simulink library "MedusaPremix"  (R2022b)
settings: Solver=VariableStepAuto  StartTime=0.0  StopTime=10.0  RelTol=1e-3
values from neighbouring files (symbols this model uses):
  PremixConfig = struct('sample_rate_in_hertz', sample_rate_in_hertz,                            'frame_size', frame_size,                            'rgain_SILENT_GAIN', rgain_SILENT_GAIN,                            'granularity', internal_granularity,                            'LR_in', LR_in, 'LR_out', LR_out,                            'CS_in', CS_in, 'CS_out', CS_out,                            'NumCenterOut' ...(+550 chars)    [MedusaPremixInit.m]
  PremixTune = MedusaPremixTuneInit(tuneFileName, headrestTuneFileName, overheadTuneFileName, MedusaParams)    [MedusaPremixInit.m]    (also in MedusaPremixTuneInit.m = load(tuneFileName))
undefined symbols (not defined in the file or in its folder): carModel, mode, MSConfig, Row
libraries: TuneVar x286, TOP x202, dspmtrx3 x146, FeaturePath x86, matrix_library x20, PooliirLib x8, Pooliir x4
(part 8 of 22)

== system MedusaPremix/Premix51WithMonoSurroundAndCae/Full Mixing Matrix_Center Surround/Fader Downmix ==
  note: downmix
  Front Fade Gain : Inport
  Back Fade Gain : Inport  Port=2
  In Bus Element : Inport  Port=3  PortName=Tuned Inputs  Element=Forward Downmix Threshold
  In Bus Element1 : Inport  Port=3  PortName=Tuned Inputs  Element=Forward Downmix Max
  In Bus Element2 : Inport  Port=3  PortName=Tuned Inputs  Element=Backward Downmix Threshold
  In Bus Element3 : Inport  Port=3  PortName=Tuned Inputs  Element=Backward Downmix Max
  In Bus Element4 : Inport  Port=3  PortName=Tuned Inputs  Element=Downmix Weights CS
  In Bus Element5 : Inport  Port=3  PortName=Tuned Inputs  Element=Downmix Weights CS CAE
  CAE_Enable : Inport  Port=4
  Trigger : TriggerPort  TriggerType=function-call  VariantControl=Variant  PortDimensions=1
  Fading Backward : Subsystem  TreatAsAtomicUnit=on
  Fading Forward : Subsystem  TreatAsAtomicUnit=on
  FeaturePath : FeaturePath/FeaturePath  FeatureName=Fade  IsGroup=off  GroupNumber=-1  DeclarePackages=off  PackageNames=mode,carModel  IsToolGroup=off  TriggerInit=[920 94 1035 201]
      settings: SourceProductName=Bose Talaria
  If : If  NumInputs=2  IfExpression=u1 >= u2
  MATLAB Function : MATLAB Function  TreatAsAtomicUnit=on
  Matrix Multiply : Product
  Merge : Merge
  Downmix : Outport  VectorParamsAs1DForOutWhenUnconnected=off
  DownmixingMatrix : Outport  Port=2  VectorParamsAs1DForOutWhenUnconnected=off
  wires:
  In Bus Element4/1 -> MATLAB Function/1(weights)
  In Bus Element5/1 -> MATLAB Function/2(weights_CAE)
  MATLAB Function/1(downmixWeights) -> Matrix Multiply/2
  In Bus Element3/1 -> Fading Backward/3(backwardDownmixMax)
  In Bus Element2/1 -> Fading Backward/2(backwardDownmixThreshold)
  In Bus Element1/1 -> Fading Forward/3(forwardDownmixMax)
  In Bus Element/1 -> Fading Forward/2(forwardDownmixThreshold)
  If/2 -> Fading Backward/Action
  Fading Forward/1(downmix) -> Merge/1
  Matrix Multiply/1 -> DownmixingMatrix/1
  Back Fade Gain/1 -> If/2, Fading Forward/1(backFadeGain)
  Merge/1 -> Downmix/1, Matrix Multiply/1
  Front Fade Gain/1 -> Fading Backward/1(frontFadeGain), If/1
  Fading Backward/1(downmix) -> Merge/2
  If/1 -> Fading Forward/Action
  CAE_Enable/1 -> MATLAB Function/3(CAE_Enable)

== system MedusaPremix/Premix51WithMonoSurroundAndCae/Full Mixing Matrix_Center Surround/Premixing ==
  Audio Channel Inputs : Inport
  Target Gain : Inport  Port=2
  Matrix Multiply1 : Product  Multiplication=Matrix(*)
  Transpose1 : Math  Operator=transpose  SignedPower=on
  Output : Outport  VectorParamsAs1DForOutWhenUnconnected=off
  wires:
  Matrix Multiply1/1 -> Output/1
  Audio Channel Inputs/1 -> Matrix Multiply1/1
  Target Gain/1 -> Transpose1/1
  Transpose1/1 -> Matrix Multiply1/2

== system MedusaPremix/Premix51WithMonoSurroundAndCae/Full Mixing Matrix_Center Surround/Surround Level Control ==
  RST Trigger : Inport
  SLC Request Trigger : Inport  Port=2
  In Bus Element : Inport  Port=3  PortName=Control Inputs  Element=surround_index
  In Bus Element1 : Inport  Port=3  PortName=Control Inputs  Element=ramp_db_per_second
  In Bus Element2 : Inport  Port=3  PortName=Control Inputs  Element=ramp_milliseconds
  Check Done : Inport  Port=4
  In Bus Element3 : Inport  Port=5  PortName=Tuned Inputs  Element=Min Level CS
  In Bus Element4 : Inport  Port=5  PortName=Tuned Inputs  Element=Detent Level CS
  In Bus Element5 : Inport  Port=5  PortName=Tuned Inputs  Element=Max Level CS
  In Bus Element6 : Inport  Port=5  PortName=Tuned Inputs  Element=Interpolation Method
  In Bus Element7 : Inport  Port=5  PortName=Tuned Inputs  Element=Min Level CS CAE
  In Bus Element8 : Inport  Port=5  PortName=Tuned Inputs  Element=Detent Level CS CAE
  In Bus Element9 : Inport  Port=5  PortName=Tuned Inputs  Element=Max Level CS CAE
  Data Store Memory3 : DataStoreMemory  DataStoreName=Premix_targetGain_CS  ReadBeforeWriteMsg=warning  WriteAfterWriteMsg=warning  WriteAfterReadMsg=warning  InitialValue=1e-5*ones(MedusaPremixConfig.CS_out,MedusaPremixConfig.CS_in)  ShowAdditionalParam=off  OutDataTypeStr=single
  Data Store Memory4 : DataStoreMemory  DataStoreName=Premix_currentGain_CS  ReadBeforeWriteMsg=warning  WriteAfterWriteMsg=warning  WriteAfterReadMsg=warning  InitialValue=1e-5*ones(MedusaPremixConfig.CS_out,MedusaPremixConfig.CS_in)  ShowAdditionalParam=off  OutDataTypeStr=single
  Data Store Read1 : DataStoreRead  DataStoreName=Premix_currentGain_CS  IndexOptions=Index vector (dialog)  Indices=1  OutputSizes=1
  FeaturePath : FeaturePath/FeaturePath  FeatureName=SLC  IsGroup=off  GroupNumber=-1  DeclarePackages=off  PackageNames=mode,carModel  IsToolGroup=off  TriggerInit=[955 319 1070 426]
      settings: SourceProductName=Bose Talaria
  Function-Call Split : FunctionCallSplit  IconShape=distinctive  NumOutputPorts=2
  Initialization and RMDL : MATLAB Function  TreatAsAtomicUnit=on
  Ramper : Subsystem
  Target Gain Computation : MATLAB Function  TreatAsAtomicUnit=on
  Gain Out : Outport  VectorParamsAs1DForOutWhenUnconnected=off
  Ramping Done : Outport  Port=2  VectorParamsAs1DForOutWhenUnconnected=off
  wires:
  In Bus Element9/1 -> Target Gain Computation/6(maxGain_CS_CAE), Initialization and RMDL/6(maxGain_CS_CAE)
  In Bus Element8/1 -> Target Gain Computation/4(detentGain_CS_CAE), Initialization and RMDL/4(detentGain_CS_CAE)
  In Bus Element7/1 -> Target Gain Computation/2(minGain_CS_CAE), Initialization and RMDL/2(minGain_CS_CAE)
  In Bus Element/1 -> Target Gain Computation/9(surr_level), Initialization and RMDL/9(surr_level)
  In Bus Element1/1 -> Ramper/3(ramp rate)
  In Bus Element2/1 -> Ramper/4(ramp time)
  In Bus Element4/1 -> Target Gain Computation/3(detentGain_CS), Initialization and RMDL/3(detentGain_CS)
  In Bus Element3/1 -> Target Gain Computation/1(minGain_CS), Initialization and RMDL/1(minGain_CS)
  In Bus Element6/1 -> Target Gain Computation/7(interpolation_method), Initialization and RMDL/7(interpolation_method)
  In Bus Element5/1 -> Target Gain Computation/5(maxGain_CS), Initialization and RMDL/5(maxGain_CS)
  Ramper/1(ramping done) -> Ramping Done/1
  SLC Request Trigger/1 -> Function-Call Split/1
  Function-Call Split/2 -> Ramper/1(RTC Recv Trigger)
  Function-Call Split/1 -> Target Gain Computation/Trigger
  Target Gain Computation/1(gain_out) -> Ramper/2(target gains (linear))
  Check Done/1 -> Ramper/5(check sequence trigger)
  RST Trigger/1 -> Initialization and RMDL/Trigger
  Data Store Read1/1 -> Gain Out/1
  [CAE_Enable] -> Initialization and RMDL/8(CAE_Enable), Target Gain Computation/8(CAE_Enable)

== system MedusaPremix/Premix51WithMonoSurroundAndCae/Full Mixing Matrix_Left/Fader Downmix ==
  note: downmix
  Front Fade Gain : Inport
  Back Fade Gain : Inport  Port=2
  In Bus Element : Inport  Port=3  PortName=Tuned Inputs  Element=Forward Downmix Threshold
  In Bus Element1 : Inport  Port=3  PortName=Tuned Inputs  Element=Forward Downmix Max
  In Bus Element2 : Inport  Port=3  PortName=Tuned Inputs  Element=Backward Downmix Threshold
  In Bus Element3 : Inport  Port=3  PortName=Tuned Inputs  Element=Backward Downmix Max
  In Bus Element4 : Inport  Port=3  PortName=Tuned Inputs  Element=Downmix Weights Left
  In Bus Element5 : Inport  Port=3  PortName=Tuned Inputs  Element=Downmix Weights Left CAE
  CAE_Enable : Inport  Port=4
  Trigger : TriggerPort  TriggerType=function-call  VariantControl=Variant  PortDimensions=1
  Fading Backward : Subsystem  TreatAsAtomicUnit=on
  Fading Forward : Subsystem  TreatAsAtomicUnit=on
  FeaturePath : FeaturePath/FeaturePath  FeatureName=Fade  IsGroup=off  GroupNumber=-1  DeclarePackages=off  PackageNames=mode,carModel  IsToolGroup=off  TriggerInit=[875 94 990 201]
      settings: SourceProductName=Bose Talaria
  If : If  NumInputs=2  IfExpression=u1 >= u2
  MATLAB Function : MATLAB Function  TreatAsAtomicUnit=on
  Matrix Multiply : Product
  Merge : Merge
  Downmix : Outport  VectorParamsAs1DForOutWhenUnconnected=off
  DownmixingMatrix : Outport  Port=2  VectorParamsAs1DForOutWhenUnconnected=off
  wires:
  In Bus Element5/1 -> MATLAB Function/2(weights_CAE)
  In Bus Element4/1 -> MATLAB Function/1(weights)
  MATLAB Function/1(downmixWeights) -> Matrix Multiply/2
  In Bus Element3/1 -> Fading Backward/3(backwardDownmixMax)
  In Bus Element2/1 -> Fading Backward/2(backwardDownmixThreshold)
  In Bus Element1/1 -> Fading Forward/3(forwardDownmixMax)
  In Bus Element/1 -> Fading Forward/2(forwardDownmixThreshold)
  If/2 -> Fading Backward/Action
  Fading Forward/1(downmix) -> Merge/1
  Matrix Multiply/1 -> DownmixingMatrix/1
  Back Fade Gain/1 -> If/2, Fading Forward/1(backFadeGain)
  Merge/1 -> Downmix/1, Matrix Multiply/1
  Front Fade Gain/1 -> Fading Backward/1(frontFadeGain), If/1
  Fading Backward/1(downmix) -> Merge/2
  If/1 -> Fading Forward/Action
  CAE_Enable/1 -> MATLAB Function/3(CAE_Enable)

== system MedusaPremix/Premix51WithMonoSurroundAndCae/Full Mixing Matrix_Left/Premixing ==
  Audio Channel Inputs : Inport
  Target Gain : Inport  Port=2
  Matrix Multiply1 : Product  Multiplication=Matrix(*)
  Transpose1 : Math  Operator=transpose  SignedPower=on
  Output : Outport  VectorParamsAs1DForOutWhenUnconnected=off
  wires:
  Matrix Multiply1/1 -> Output/1
  Audio Channel Inputs/1 -> Matrix Multiply1/1
  Target Gain/1 -> Transpose1/1
  Transpose1/1 -> Matrix Multiply1/2

== system MedusaPremix/Premix51WithMonoSurroundAndCae/Full Mixing Matrix_Left/Surround Level Control ==
  RST Trigger : Inport
  SLC Request Trigger : Inport  Port=2
  In Bus Element : Inport  Port=3  PortName=Control Inputs  Element=surround_index
  In Bus Element1 : Inport  Port=3  PortName=Control Inputs  Element=ramp_db_per_second
  In Bus Element2 : Inport  Port=3  PortName=Control Inputs  Element=ramp_milliseconds
  Check Done : Inport  Port=4
  In Bus Element3 : Inport  Port=5  PortName=Tuned Inputs  Element=Min Level Left
  In Bus Element4 : Inport  Port=5  PortName=Tuned Inputs  Element=Detent Level Left
  In Bus Element5 : Inport  Port=5  PortName=Tuned Inputs  Element=Max Level Left
  In Bus Element6 : Inport  Port=5  PortName=Tuned Inputs  Element=Interpolation Method
  In Bus Element7 : Inport  Port=5  PortName=Tuned Inputs  Element=Min Level Left CAE
  In Bus Element8 : Inport  Port=5  PortName=Tuned Inputs  Element=Detent Level Left CAE
  In Bus Element9 : Inport  Port=5  PortName=Tuned Inputs  Element=Max Level Left CAE
  Data Store Memory3 : DataStoreMemory  DataStoreName=Premix_targetGain_Left  ReadBeforeWriteMsg=warning  WriteAfterWriteMsg=warning  WriteAfterReadMsg=warning  InitialValue=1e-5*ones(MedusaPremixConfig.LR_out,MedusaPremixConfig.LR_in)  ShowAdditionalParam=off  OutDataTypeStr=single
  Data Store Memory4 : DataStoreMemory  DataStoreName=Premix_currentGain_Left  ReadBeforeWriteMsg=warning  WriteAfterWriteMsg=warning  WriteAfterReadMsg=warning  InitialValue=1e-5*ones(MedusaPremixConfig.LR_out,MedusaPremixConfig.LR_in)  ShowAdditionalParam=off  OutDataTypeStr=single
  Data Store Read1 : DataStoreRead  DataStoreName=Premix_currentGain_Left  IndexOptions=Index vector (dialog)  Indices=1  OutputSizes=1
  FeaturePath : FeaturePath/FeaturePath  FeatureName=SLC  IsGroup=off  GroupNumber=-1  DeclarePackages=off  PackageNames=mode,carModel  IsToolGroup=off  TriggerInit=[955 384 1070 491]
      settings: SourceProductName=Bose Talaria
  Function-Call Split : FunctionCallSplit  IconShape=distinctive  NumOutputPorts=2
  Initialization and RMDL : MATLAB Function  TreatAsAtomicUnit=on
  Ramper : Subsystem
  Target Gain Computation : MATLAB Function  TreatAsAtomicUnit=on
  Gain Out : Outport  VectorParamsAs1DForOutWhenUnconnected=off
  Ramping Done : Outport  Port=2  VectorParamsAs1DForOutWhenUnconnected=off
  wires:
  In Bus Element7/1 -> Target Gain Computation/2(minGain_Left_CAE), Initialization and RMDL/2(minGain_Left_CAE)
  In Bus Element8/1 -> Target Gain Computation/4(detentGain_Left_CAE), Initialization and RMDL/4(detentGain_Left_CAE)
  In Bus Element9/1 -> Target Gain Computation/6(maxGain_Left_CAE), Initialization and RMDL/6(maxGain_Left_CAE)
  In Bus Element4/1 -> Target Gain Computation/3(detentGain_Left), Initialization and RMDL/3(detentGain_Left)
  In Bus Element3/1 -> Target Gain Computation/1(minGain_Left), Initialization and RMDL/1(minGain_Left)
  In Bus Element6/1 -> Target Gain Computation/7(interpolation_method), Initialization and RMDL/7(interpolation_method)
  In Bus Element5/1 -> Target Gain Computation/5(maxGain_Left), Initialization and RMDL/5(maxGain_Left)
  Ramper/1(ramping done) -> Ramping Done/1
  SLC Request Trigger/1 -> Function-Call Split/1
  Function-Call Split/2 -> Ramper/1(RTC Recv Trigger)
  Function-Call Split/1 -> Target Gain Computation/Trigger
  Target Gain Computation/1(gain_out) -> Ramper/2(target gains (linear))
  Check Done/1 -> Ramper/5(check sequence trigger)
  RST Trigger/1 -> Initialization and RMDL/Trigger
  Data Store Read1/1 -> Gain Out/1
  In Bus Element/1 -> Target Gain Computation/9(surr_level), Initialization and RMDL/9(surr_level)
  In Bus Element1/1 -> Ramper/3(ramp rate)
  In Bus Element2/1 -> Ramper/4(ramp time)
  [CAE_Enable] -> Target Gain Computation/8(CAE_Enable), Initialization and RMDL/8(CAE_Enable)

== system MedusaPremix/Premix51WithMonoSurroundAndCae/Full Mixing Matrix_Right/Fader Downmix ==
  note: downmix
  Front Fade Gain : Inport
  Back Fade Gain : Inport  Port=2
  In Bus Element : Inport  Port=3  PortName=Tuned Inputs  Element=Forward Downmix Threshold
  In Bus Element1 : Inport  Port=3  PortName=Tuned Inputs  Element=Forward Downmix Max
  In Bus Element2 : Inport  Port=3  PortName=Tuned Inputs  Element=Backward Downmix Threshold
  In Bus Element3 : Inport  Port=3  PortName=Tuned Inputs  Element=Backward Downmix Max
  In Bus Element4 : Inport  Port=3  PortName=Tuned Inputs  Element=Downmix Weights Right
  In Bus Element5 : Inport  Port=3  PortName=Tuned Inputs  Element=Downmix Weights Right CAE
  CAE_Enable : Inport  Port=4
  Trigger : TriggerPort  TriggerType=function-call  VariantControl=Variant  PortDimensions=1
  Fading Backward : Subsystem  TreatAsAtomicUnit=on
  Fading Forward : Subsystem  TreatAsAtomicUnit=on
  FeaturePath : FeaturePath/FeaturePath  FeatureName=Fade  IsGroup=off  GroupNumber=-1  DeclarePackages=off  PackageNames=mode,carModel  IsToolGroup=off  TriggerInit=[875 94 990 201]
      settings: SourceProductName=Bose Talaria
  If : If  NumInputs=2  IfExpression=u1 >= u2
  MATLAB Function : MATLAB Function  TreatAsAtomicUnit=on
  Matrix Multiply : Product
  Merge : Merge
  Downmix : Outport  VectorParamsAs1DForOutWhenUnconnected=off
  DownmixingMatrix : Outport  Port=2  VectorParamsAs1DForOutWhenUnconnected=off
  wires:
  In Bus Element4/1 -> MATLAB Function/1(weights)
  In Bus Element5/1 -> MATLAB Function/2(weights_CAE)
  MATLAB Function/1(downmixWeights) -> Matrix Multiply/2
  In Bus Element3/1 -> Fading Backward/3(backwardDownmixMax)
  In Bus Element2/1 -> Fading Backward/2(backwardDownmixThreshold)
  In Bus Element1/1 -> Fading Forward/3(forwardDownmixMax)
  In Bus Element/1 -> Fading Forward/2(forwardDownmixThreshold)
  If/2 -> Fading Backward/Action
  Fading Forward/1(downmix) -> Merge/1
  Matrix Multiply/1 -> DownmixingMatrix/1
  Back Fade Gain/1 -> If/2, Fading Forward/1(backFadeGain)
  Merge/1 -> Downmix/1, Matrix Multiply/1
  Front Fade Gain/1 -> Fading Backward/1(frontFadeGain), If/1
  Fading Backward/1(downmix) -> Merge/2
  If/1 -> Fading Forward/Action
  CAE_Enable/1 -> MATLAB Function/3(CAE_Enable)

== system MedusaPremix/Premix51WithMonoSurroundAndCae/Full Mixing Matrix_Right/Premixing ==
  Audio Channel Inputs : Inport
  Target Gain : Inport  Port=2
  Matrix Multiply1 : Product  Multiplication=Matrix(*)
  Transpose1 : Math  Operator=transpose  SignedPower=on
  Output : Outport  VectorParamsAs1DForOutWhenUnconnected=off
  wires:
  Matrix Multiply1/1 -> Output/1
  Audio Channel Inputs/1 -> Matrix Multiply1/1
  Target Gain/1 -> Transpose1/1
  Transpose1/1 -> Matrix Multiply1/2

== system MedusaPremix/Premix51WithMonoSurroundAndCae/Full Mixing Matrix_Right/Surround Level Control ==
  RST Trigger : Inport
  SLC Request Trigger : Inport  Port=2
  In Bus Element : Inport  Port=3  PortName=Control Inputs  Element=surround_index
  In Bus Element1 : Inport  Port=3  PortName=Control Inputs  Element=ramp_db_per_second
  In Bus Element2 : Inport  Port=3  PortName=Control Inputs  Element=ramp_milliseconds
  Check Done : Inport  Port=4
  In Bus Element3 : Inport  Port=5  PortName=Tuned Inputs  Element=Min Level Right
  In Bus Element4 : Inport  Port=5  PortName=Tuned Inputs  Element=Detent Level Right
  In Bus Element5 : Inport  Port=5  PortName=Tuned Inputs  Element=Max Level Right
  In Bus Element7 : Inport  Port=5  PortName=Tuned Inputs  Element=Interpolation Method
  In Bus Element6 : Inport  Port=5  PortName=Tuned Inputs  Element=Min Level Right CAE
  In Bus Element8 : Inport  Port=5  PortName=Tuned Inputs  Element=Detent Level Right CAE
  In Bus Element9 : Inport  Port=5  PortName=Tuned Inputs  Element=Max Level Right CAE
  Data Store Memory3 : DataStoreMemory  DataStoreName=Premix_targetGain_Right  ReadBeforeWriteMsg=warning  WriteAfterWriteMsg=warning  WriteAfterReadMsg=warning  InitialValue=1e-5*ones(MedusaPremixConfig.LR_out,MedusaPremixConfig.LR_in)  ShowAdditionalParam=off  OutDataTypeStr=single
  Data Store Memory4 : DataStoreMemory  DataStoreName=Premix_currentGain_Right  ReadBeforeWriteMsg=warning  WriteAfterWriteMsg=warning  WriteAfterReadMsg=warning  InitialValue=1e-5*ones(MedusaPremixConfig.LR_out,MedusaPremixConfig.LR_in)  ShowAdditionalParam=off  OutDataTypeStr=single
  Data Store Read1 : DataStoreRead  DataStoreName=Premix_currentGain_Right  IndexOptions=Index vector (dialog)  Indices=1  OutputSizes=1
  FeaturePath : FeaturePath/FeaturePath  FeatureName=SLC  IsGroup=off  GroupNumber=-1  DeclarePackages=off  PackageNames=mode,carModel  IsToolGroup=off  TriggerInit=[955 319 1070 426]
      settings: SourceProductName=Bose Talaria
  Function-Call Split : FunctionCallSplit  IconShape=distinctive  NumOutputPorts=2
  Initialization and RMDL : MATLAB Function  TreatAsAtomicUnit=on
  Ramper : Subsystem
  Target Gain Computation : MATLAB Function  TreatAsAtomicUnit=on
  Gain Out : Outport  VectorParamsAs1DForOutWhenUnconnected=off
  Ramping Done : Outport  Port=2  VectorParamsAs1DForOutWhenUnconnected=off
  wires:
  In Bus Element4/1 -> Initialization and RMDL/3(detentGain_Right), Target Gain Computation/3(detentGain_Right)
  In Bus Element6/1 -> Initialization and RMDL/2(minGain_Right_CAE), Target Gain Computation/2(minGain_Right_CAE)
  In Bus Element8/1 -> Initialization and RMDL/4(detentGain_Right_CAE), Target Gain Computation/4(detentGain_Right_CAE)
  In Bus Element9/1 -> Initialization and RMDL/6(maxGain_Right_CAE), Target Gain Computation/6(maxGain_Right_CAE)
  In Bus Element/1 -> Target Gain Computation/9(surr_level), Initialization and RMDL/9(surr_level)
  In Bus Element1/1 -> Ramper/3(ramp rate)
  In Bus Element2/1 -> Ramper/4(ramp time)
  In Bus Element3/1 -> Initialization and RMDL/1(minGain_Right), Target Gain Computation/1(minGain_Right)
  In Bus Element7/1 -> Initialization and RMDL/7(interpolation_method), Target Gain Computation/7(interpolation_method)
  In Bus Element5/1 -> Initialization and RMDL/5(maxGain_Right), Target Gain Computation/5(maxGain_Right)
  Ramper/1(ramping done) -> Ramping Done/1
  SLC Request Trigger/1 -> Function-Call Split/1
  Function-Call Split/2 -> Ramper/1(RTC Recv Trigger)
  Function-Call Split/1 -> Target Gain Computation/Trigger
  Target Gain Computation/1(gain_out) -> Ramper/2(target gains (linear))
  Check Done/1 -> Ramper/5(check sequence trigger)
  RST Trigger/1 -> Initialization and RMDL/Trigger
  Data Store Read1/1 -> Gain Out/1
  [CAE_Enable] -> Target Gain Computation/8(CAE_Enable), Initialization and RMDL/8(CAE_Enable)

== system MedusaPremix/Premix51WithMonoSurroundAndCae/Input Organizer/Bass Component Splitter ==
  Bass Inputs : Inport
  Submatrix : dspmtrx3/Submatrix  RowSpan=All rows  RowStartMode=First  RowStartIndex=1  RowEndMode=Last  RowEndIndex=1  ColSpan=One column  ColStartMode=First  ColStartIndex=1  ColEndMode=Last  ColEndIndex=1
  Submatrix1 : dspmtrx3/Submatrix  RowSpan=All rows  RowStartMode=First  RowStartIndex=1  RowEndMode=Last  RowEndIndex=1  ColSpan=One column  ColStartMode=Last  ColStartIndex=1  ColEndMode=Last  ColEndIndex=1
  Lbass : Outport  VectorParamsAs1DForOutWhenUnconnected=off
  Rbass : Outport  Port=2  VectorParamsAs1DForOutWhenUnconnected=off
  wires:
  Submatrix1/1 -> Rbass/1
  Bass Inputs/1 -> Submatrix/1, Submatrix1/1
  Submatrix/1 -> Lbass/1

== system MedusaPremix/Premix51WithMonoSurroundAndCae/Input Organizer/Discrete Surround Component Splitter ==
  Discrete Surround Inputs : Inport
  Submatrix : dspmtrx3/Submatrix  RowSpan=All rows  RowStartMode=First  RowStartIndex=1  RowEndMode=Last  RowEndIndex=1  ColSpan=One column  ColStartMode=First  ColStartIndex=1  ColEndMode=Last  ColEndIndex=1
  Submatrix1 : dspmtrx3/Submatrix  RowSpan=All rows  RowStartMode=First  RowStartIndex=1  RowEndMode=Last  RowEndIndex=1  ColSpan=One column  ColStartMode=Middle  ColStartIndex=1  ColEndMode=Last  ColEndIndex=1
  Submatrix2 : dspmtrx3/Submatrix  RowSpan=All rows  RowStartMode=First  RowStartIndex=1  RowEndMode=Last  RowEndIndex=1  ColSpan=One column  ColStartMode=Last  ColStartIndex=3  ColEndMode=Last  ColEndIndex=1
  Ci : Outport  VectorParamsAs1DForOutWhenUnconnected=off
  Lsi : Outport  Port=2  VectorParamsAs1DForOutWhenUnconnected=off
  Rsi : Outport  Port=3  VectorParamsAs1DForOutWhenUnconnected=off
  wires:
  Submatrix/1 -> Ci/1
  Submatrix1/1 -> Lsi/1
  Submatrix2/1 -> Rsi/1
  Discrete Surround Inputs/1 -> Submatrix/1, Submatrix2/1, Submatrix1/1

== system MedusaPremix/Premix51WithMonoSurroundAndCae/Input Organizer/Mid-Range Component Splitter ==
  Mid-Range I/P : Inport
  Submatrix1 : dspmtrx3/Submatrix  RowSpan=All rows  RowStartMode=First  RowStartIndex=1  RowEndMode=Last  RowEndIndex=1  ColSpan=One column  ColStartMode=Index  ColStartIndex=7  ColEndMode=Last  ColEndIndex=1
  Submatrix2 : dspmtrx3/Submatrix  RowSpan=All rows  RowStartMode=First  RowStartIndex=1  RowEndMode=Last  RowEndIndex=1  ColSpan=One column  ColStartMode=Index  ColStartIndex=1  ColEndMode=Last  ColEndIndex=1
  Submatrix3 : dspmtrx3/Submatrix  RowSpan=All rows  RowStartMode=First  RowStartIndex=1  RowEndMode=Last  RowEndIndex=1  ColSpan=One column  ColStartMode=Index  ColStartIndex=2  ColEndMode=Last  ColEndIndex=1
  Submatrix4 : dspmtrx3/Submatrix  RowSpan=All rows  RowStartMode=First  RowStartIndex=1  RowEndMode=Last  RowEndIndex=1  ColSpan=One column  ColStartMode=Index  ColStartIndex=3  ColEndMode=Last  ColEndIndex=1
  Submatrix5 : dspmtrx3/Submatrix  RowSpan=All rows  RowStartMode=First  RowStartIndex=1  RowEndMode=Last  RowEndIndex=1  ColSpan=One column  ColStartMode=Index  ColStartIndex=4  ColEndMode=Last  ColEndIndex=1
  Submatrix6 : dspmtrx3/Submatrix  RowSpan=All rows  RowStartMode=First  RowStartIndex=1  RowEndMode=Last  RowEndIndex=1  ColSpan=One column  ColStartMode=Index  ColStartIndex=5  ColEndMode=Last  ColEndIndex=1
  Submatrix7 : dspmtrx3/Submatrix  RowSpan=All rows  RowStartMode=First  RowStartIndex=1  RowEndMode=Last  RowEndIndex=1  ColSpan=One column  ColStartMode=Index  ColStartIndex=6  ColEndMode=Last  ColEndIndex=1
  Submatrix8 : dspmtrx3/Submatrix  RowSpan=All rows  RowStartMode=First  RowStartIndex=1  RowEndMode=Last  RowEndIndex=1  ColSpan=One column  ColStartMode=Index  ColStartIndex=8  ColEndMode=Last  ColEndIndex=1
  Lo : Outport  VectorParamsAs1DForOutWhenUnconnected=off
  Ro : Outport  Port=2  VectorParamsAs1DForOutWhenUnconnected=off
  Ls : Outport  Port=3  VectorParamsAs1DForOutWhenUnconnected=off
  Rs : Outport  Port=4  VectorParamsAs1DForOutWhenUnconnected=off
  Limp : Outport  Port=5  VectorParamsAs1DForOutWhenUnconnected=off
  Ltail : Outport  Port=6  VectorParamsAs1DForOutWhenUnconnected=off
  Rimp : Outport  Port=7  VectorParamsAs1DForOutWhenUnconnected=off
  Rtail : Outport  Port=8  VectorParamsAs1DForOutWhenUnconnected=off
  wires:
  Submatrix3/1 -> Ro/1
  Submatrix2/1 -> Lo/1
  Submatrix4/1 -> Ls/1
  Submatrix5/1 -> Rs/1
  Submatrix7/1 -> Ltail/1
  Submatrix6/1 -> Limp/1
  Submatrix8/1 -> Rtail/1
  Submatrix1/1 -> Rimp/1
  Mid-Range I/P/1 -> Submatrix1/1, Submatrix8/1, Submatrix7/1, Submatrix2/1, Submatrix3/1, Submatrix4/1, Submatrix5/1, Submatrix6/1

== system MedusaPremix/Premix51WithMonoSurroundAndCae/Input Organizer/Wiggle Component Splitter ==
  Wiggle Filter O/P : Inport
  Submatrix : dspmtrx3/Submatrix  RowSpan=All rows  RowStartMode=First  RowStartIndex=1  RowEndMode=Last  RowEndIndex=1  ColSpan=One column  ColStartMode=Index  ColStartIndex=1  ColEndMode=Last  ColEndIndex=1
  Submatrix1 : dspmtrx3/Submatrix  RowSpan=All rows  RowStartMode=First  RowStartIndex=1  RowEndMode=Last  RowEndIndex=1  ColSpan=One column  ColStartMode=Index  ColStartIndex=2  ColEndMode=Last  ColEndIndex=1
  Submatrix2 : dspmtrx3/Submatrix  RowSpan=All rows  RowStartMode=First  RowStartIndex=1  RowEndMode=Last  RowEndIndex=1  ColSpan=One column  ColStartMode=Index  ColStartIndex=3  ColEndMode=Last  ColEndIndex=1
  Submatrix3 : dspmtrx3/Submatrix  RowSpan=All rows  RowStartMode=First  RowStartIndex=1  RowEndMode=Last  RowEndIndex=1  ColSpan=One column  ColStartMode=Index  ColStartIndex=4  ColEndMode=Last  ColEndIndex=1
  Lftail : Outport  VectorParamsAs1DForOutWhenUnconnected=off
  Lrtail : Outport  Port=2  VectorParamsAs1DForOutWhenUnconnected=off
  Rftail : Outport  Port=3  VectorParamsAs1DForOutWhenUnconnected=off
  Rrtail : Outport  Port=4  VectorParamsAs1DForOutWhenUnconnected=off
  wires:
  Submatrix3/1 -> Rrtail/1
  Submatrix/1 -> Lftail/1
  Wiggle Filter O/P/1 -> Submatrix3/1, Submatrix2/1, Submatrix1/1, Submatrix/1
  Submatrix2/1 -> Lrtail/1
  Submatrix1/1 -> Rftail/1

== system MedusaPremix/Premix51WithMonoSurroundAndCae/SLC Tuning/Detent Level CS ==
  TOP : TOP/TOP  TriggerInit=[440 -15 585 45]  TopName=DetentLevel_CS  DataType=single  BankNumber=0  Role=Automatic
      settings: SourceProductName=Bose Talaria
  TOP1 : TOP/TOP  TriggerInit=[440 55 585 115]  TopName=DetentLevel_CS_CAE  DataType=single  BankNumber=0  Role=Automatic
      settings: SourceProductName=Bose Talaria
  TranslateTrigger : TuneVar/TranslateTrigger  TriggerInit=[306 -100 344 -45]
      settings: SourceProductName=Bose Talaria
  Trivial Translation : MATLAB Function  TreatAsAtomicUnit=on
  Tune Variable : TuneVar/Tune Variable  TuneName=DetentLevel_CS  SpecifyMaxSize=off  VariableDim=1 (Row)  MaxSize=[1 1]  PackageName=mode  TunabilityNumber=1  MinValue=[0]  MaxValue=[1]  TriggerInit=[-35 25 135 75]  MaskValue=MedusaPremixTune.detentGain_CS
      settings: SourceProductName=Bose Talaria
  Out1 : Outport  VectorParamsAs1DForOutWhenUnconnected=off
  Out2 : Outport  Port=2  VectorParamsAs1DForOutWhenUnconnected=off
  wires:
  TOP/1 -> Out1/1  "DetentLevel_CS"
  Tune Variable/1 -> Trivial Translation/1(detentGain_CS)  "DetentLevel_CS"
  Trivial Translation/1(TOP) -> TOP/1
  TranslateTrigger/1 -> Trivial Translation/Trigger
  TOP1/1 -> Out2/1  "DetentLevel_CS_CAE"
  Trivial Translation/2(TOP_CAE) -> TOP1/1

== system MedusaPremix/Premix51WithMonoSurroundAndCae/SLC Tuning/Detent Level Left ==
  TOP : TOP/TOP  TriggerInit=[440 -15 585 45]  TopName=DetentLevel_Left  DataType=single  BankNumber=0  Role=Automatic
      settings: SourceProductName=Bose Talaria
  TOP1 : TOP/TOP  TriggerInit=[440 55 585 115]  TopName=DetentLevel_Left_CAE  DataType=single  BankNumber=0  Role=Automatic
      settings: SourceProductName=Bose Talaria
  TranslateTrigger : TuneVar/TranslateTrigger  TriggerInit=[306 -100 344 -45]
      settings: SourceProductName=Bose Talaria
  Trivial Translation : MATLAB Function  TreatAsAtomicUnit=on
  Tune Variable : TuneVar/Tune Variable  TuneName=DetentLevel_Left  SpecifyMaxSize=off  VariableDim=1 (Row)  MaxSize=[1 1]  PackageName=mode  TunabilityNumber=1  MinValue=[0]  MaxValue=[1]  TriggerInit=[-65 25 105 75]  MaskValue=MedusaPremixTune.detentGain_Left
      settings: SourceProductName=Bose Talaria
  Out1 : Outport  VectorParamsAs1DForOutWhenUnconnected=off
  Out2 : Outport  Port=2  VectorParamsAs1DForOutWhenUnconnected=off
  wires:
  TOP/1 -> Out1/1  "DetentLevel_Left"
  Tune Variable/1 -> Trivial Translation/1(detentGain_Left)  "DetentLevel_Left"
  Trivial Translation/1(TOP) -> TOP/1
  TranslateTrigger/1 -> Trivial Translation/Trigger
  TOP1/1 -> Out2/1  "DetentLevel_Left_CAE"
  Trivial Translation/2(TOP_CAE) -> TOP1/1

== system MedusaPremix/Premix51WithMonoSurroundAndCae/SLC Tuning/Detent Level Right ==
  TOP : TOP/TOP  TriggerInit=[440 -15 585 45]  TopName=DetentLevel_Right  DataType=single  BankNumber=0  Role=Automatic
      settings: SourceProductName=Bose Talaria
  TOP1 : TOP/TOP  TriggerInit=[440 55 585 115]  TopName=DetentLevel_Right_CAE  DataType=single  BankNumber=0  Role=Automatic
      settings: SourceProductName=Bose Talaria
  TranslateTrigger : TuneVar/TranslateTrigger  TriggerInit=[306 -100 344 -45]
      settings: SourceProductName=Bose Talaria
  Trivial Translation : MATLAB Function  TreatAsAtomicUnit=on
  Tune Variable : TuneVar/Tune Variable  TuneName=DetentLevel_Right  SpecifyMaxSize=off  VariableDim=1 (Row)  MaxSize=[1 1]  PackageName=mode  TunabilityNumber=1  MinValue=[0]  MaxValue=[1]  TriggerInit=[-60 25 110 75]  MaskValue=MedusaPremixTune.detentGain_Right
      settings: SourceProductName=Bose Talaria
  Out1 : Outport  VectorParamsAs1DForOutWhenUnconnected=off
  Out2 : Outport  Port=2  VectorParamsAs1DForOutWhenUnconnected=off
  wires:
  TOP/1 -> Out1/1  "DetentLevel_Right"
  Tune Variable/1 -> Trivial Translation/1(detentGain_Right)  "DetentLevel_Right"
  Trivial Translation/1(TOP) -> TOP/1
  TranslateTrigger/1 -> Trivial Translation/Trigger
  TOP1/1 -> Out2/1  "DetentLevel_Right_CAE"
  Trivial Translation/2(TOP_CAE) -> TOP1/1

== system MedusaPremix/Premix51WithMonoSurroundAndCae/SLC Tuning/Interpolation Method ==
  TOP : TOP/TOP  TriggerInit=[440 20 585 80]  TopName=Interpolation_Method  DataType=single  BankNumber=0  Role=Automatic
      settings: SourceProductName=Bose Talaria
  TranslateTrigger : TuneVar/TranslateTrigger  TriggerInit=[306 -100 344 -45]
      settings: SourceProductName=Bose Talaria
  Trivial Translation : MATLAB Function  TreatAsAtomicUnit=on
  Tune Variable : TuneVar/Tune Variable  TuneName=Interpolation_Method  SpecifyMaxSize=off  VariableDim=1 (Row)  MaxSize=[1 1]  PackageName=mode  TunabilityNumber=2  MinValue=[0]  MaxValue=[1]  TriggerInit=[-40 25 130 75]  MaskValue=MedusaPremixTune.interpolationMethod
      settings: SourceProductName=Bose Talaria
  Out1 : Outport  VectorParamsAs1DForOutWhenUnconnected=off
  wires:
  TOP/1 -> Out1/1  "Interpolation_Method"
  Tune Variable/1 -> Trivial Translation/1(interpolationMethod)  "Interpolation_Method"
  Trivial Translation/1(TOP) -> TOP/1
  TranslateTrigger/1 -> Trivial Translation/Trigger

== system MedusaPremix/Premix51WithMonoSurroundAndCae/SLC Tuning/Max Level CS ==
  TOP : TOP/TOP  TriggerInit=[440 -15 585 45]  TopName=MaxLevel_CS  DataType=single  BankNumber=0  Role=Automatic
      settings: SourceProductName=Bose Talaria
  TOP1 : TOP/TOP  TriggerInit=[440 55 585 115]  TopName=MaxLevel_CS_CAE  DataType=single  BankNumber=0  Role=Automatic
      settings: SourceProductName=Bose Talaria
  TranslateTrigger : TuneVar/TranslateTrigger  TriggerInit=[306 -100 344 -45]
      settings: SourceProductName=Bose Talaria
  Trivial Translation : MATLAB Function  TreatAsAtomicUnit=on
  Tune Variable : TuneVar/Tune Variable  TuneName=MaxLevel_CS  SpecifyMaxSize=off  VariableDim=1 (Row)  MaxSize=[1 1]  PackageName=mode  TunabilityNumber=1  MinValue=[0]  MaxValue=[1]  TriggerInit=[-45 25 125 75]  MaskValue=MedusaPremixTune.maxGain_CS
      settings: SourceProductName=Bose Talaria
  Out1 : Outport  VectorParamsAs1DForOutWhenUnconnected=off
  Out2 : Outport  Port=2  VectorParamsAs1DForOutWhenUnconnected=off
  wires:
  TOP/1 -> Out1/1  "MaxLevel_CS"
  Tune Variable/1 -> Trivial Translation/1(maxGain_CS)  "MaxLevel_CS"
  Trivial Translation/1(TOP) -> TOP/1
  TranslateTrigger/1 -> Trivial Translation/Trigger
  TOP1/1 -> Out2/1  "MaxLevel_CS_CAE"
  Trivial Translation/2(TOP_CAE) -> TOP1/1

== system MedusaPremix/Premix51WithMonoSurroundAndCae/SLC Tuning/Max Level Left ==
  TOP : TOP/TOP  TriggerInit=[440 -15 585 45]  TopName=MaxLevel_Left  DataType=single  BankNumber=0  Role=Automatic
      settings: SourceProductName=Bose Talaria
  TOP1 : TOP/TOP  TriggerInit=[440 55 585 115]  TopName=MaxLevel_Left_CAE  DataType=single  BankNumber=0  Role=Automatic
      settings: SourceProductName=Bose Talaria
  TranslateTrigger : TuneVar/TranslateTrigger  TriggerInit=[306 -100 344 -45]
      settings: SourceProductName=Bose Talaria
  Trivial Translation : MATLAB Function  TreatAsAtomicUnit=on
  Tune Variable : TuneVar/Tune Variable  TuneName=MaxLevel_Left  SpecifyMaxSize=off  VariableDim=1 (Row)  MaxSize=[1 1]  PackageName=mode  TunabilityNumber=1  MinValue=[0]  MaxValue=[1]  TriggerInit=[-55 25 115 75]  MaskValue=MedusaPremixTune.maxGain_Left
      settings: SourceProductName=Bose Talaria
  Out1 : Outport  VectorParamsAs1DForOutWhenUnconnected=off
  Out2 : Outport  Port=2  VectorParamsAs1DForOutWhenUnconnected=off
  wires:
  TOP/1 -> Out1/1  "MaxLevel_Left"
  Tune Variable/1 -> Trivial Translation/1(maxGain_Left)  "MaxLevel_Left"
  Trivial Translation/1(TOP) -> TOP/1
  TranslateTrigger/1 -> Trivial Translation/Trigger
  TOP1/1 -> Out2/1  "MaxLevel_Left_CAE"
  Trivial Translation/2(TOP_CAE) -> TOP1/1

== system MedusaPremix/Premix51WithMonoSurroundAndCae/SLC Tuning/Max Level Right ==
  TOP : TOP/TOP  TriggerInit=[440 -15 585 45]  TopName=MaxLevel_Right  DataType=single  BankNumber=0  Role=Automatic
      settings: SourceProductName=Bose Talaria
  TOP1 : TOP/TOP  TriggerInit=[440 55 585 115]  TopName=MaxLevel_Right_CAE  DataType=single  BankNumber=0  Role=Automatic
      settings: SourceProductName=Bose Talaria
  TranslateTrigger : TuneVar/TranslateTrigger  TriggerInit=[306 -100 344 -45]
      settings: SourceProductName=Bose Talaria
  Trivial Translation : MATLAB Function  TreatAsAtomicUnit=on
  Tune Variable : TuneVar/Tune Variable  TuneName=MaxLevel_Right  SpecifyMaxSize=off  VariableDim=1 (Row)  MaxSize=[1 1]  PackageName=mode  TunabilityNumber=1  MinValue=[0]  MaxValue=[1]  TriggerInit=[-40 25 130 75]  MaskValue=MedusaPremixTune.maxGain_Right
      settings: SourceProductName=Bose Talaria
  Out1 : Outport  VectorParamsAs1DForOutWhenUnconnected=off
  Out2 : Outport  Port=2  VectorParamsAs1DForOutWhenUnconnected=off
  wires:
  TOP/1 -> Out1/1  "MaxLevel_Right"
  Tune Variable/1 -> Trivial Translation/1(maxGain_Right)  "MaxLevel_Right"
  Trivial Translation/1(TOP) -> TOP/1
  TranslateTrigger/1 -> Trivial Translation/Trigger
  TOP1/1 -> Out2/1  "MaxLevel_Right_CAE"
  Trivial Translation/2(TOP_CAE) -> TOP1/1

== system MedusaPremix/Premix51WithMonoSurroundAndCae/SLC Tuning/Min Level CS ==
  TOP : TOP/TOP  TriggerInit=[440 -15 585 45]  TopName=MinLevel_CS  DataType=single  BankNumber=0  Role=Automatic
      settings: SourceProductName=Bose Talaria
  TOP1 : TOP/TOP  TriggerInit=[440 55 585 115]  TopName=MinLevel_CS_CAE  DataType=single  BankNumber=0  Role=Automatic
      settings: SourceProductName=Bose Talaria
  TranslateTrigger : TuneVar/TranslateTrigger  TriggerInit=[306 -100 344 -45]
      settings: SourceProductName=Bose Talaria
  Trivial Translation : MATLAB Function  TreatAsAtomicUnit=on
  Tune Variable : TuneVar/Tune Variable  TuneName=MinLevel_CS  SpecifyMaxSize=off  VariableDim=1 (Row)  MaxSize=[1 1]  PackageName=mode  TunabilityNumber=1  MinValue=[0]  MaxValue=[1]  TriggerInit=[-45 25 125 75]  MaskValue=MedusaPremixTune.minGain_CS
      settings: SourceProductName=Bose Talaria
  Out1 : Outport  VectorParamsAs1DForOutWhenUnconnected=off
  Out2 : Outport  Port=2  VectorParamsAs1DForOutWhenUnconnected=off
  wires:
  TOP/1 -> Out1/1  "MinLevel_CS"
  Tune Variable/1 -> Trivial Translation/1(minGain_CS)  "MinLevel_CS"
  Trivial Translation/1(TOP) -> TOP/1
  TranslateTrigger/1 -> Trivial Translation/Trigger
  TOP1/1 -> Out2/1  "MinLevel_CS_CAE"
  Trivial Translation/2(TOP_CAE) -> TOP1/1

== system MedusaPremix/Premix51WithMonoSurroundAndCae/SLC Tuning/Min Level Left ==
  TOP : TOP/TOP  TriggerInit=[380 -20 525 40]  TopName=MinLevel_Left  DataType=single  BankNumber=0  Role=Automatic
      settings: SourceProductName=Bose Talaria
  TOP1 : TOP/TOP  TriggerInit=[380 50 525 110]  TopName=MinLevel_Left_CAE  DataType=single  BankNumber=0  Role=Automatic
      settings: SourceProductName=Bose Talaria
  TranslateTrigger : TuneVar/TranslateTrigger  TriggerInit=[246 -105 284 -50]
      settings: SourceProductName=Bose Talaria
  Trivial Translation : MATLAB Function  TreatAsAtomicUnit=on
  Tune Variable : TuneVar/Tune Variable  TuneName=MinLevel_Left  SpecifyMaxSize=off  VariableDim=1 (Row)  MaxSize=[1 1]  PackageName=mode  TunabilityNumber=1  MinValue=[0]  MaxValue=[1]  TriggerInit=[-120 20 50 70]  MaskValue=MedusaPremixTune.minGain_Left
      settings: SourceProductName=Bose Talaria
  Out1 : Outport  VectorParamsAs1DForOutWhenUnconnected=off
  Out2 : Outport  Port=2  VectorParamsAs1DForOutWhenUnconnected=off
  wires:
  TOP/1 -> Out1/1  "MinLevel_Left"
  Tune Variable/1 -> Trivial Translation/1(minGain_Left)  "MinLevel_Left"
  Trivial Translation/1(TOP) -> TOP/1
  TranslateTrigger/1 -> Trivial Translation/Trigger
  TOP1/1 -> Out2/1  "MinLevel_Left_CAE"
  Trivial Translation/2(TOP_CAE) -> TOP1/1

== system MedusaPremix/Premix51WithMonoSurroundAndCae/SLC Tuning/Min Level Right ==
  TOP : TOP/TOP  TriggerInit=[440 -15 585 45]  TopName=MinLevel_Right  DataType=single  BankNumber=0  Role=Automatic
      settings: SourceProductName=Bose Talaria
  TOP1 : TOP/TOP  TriggerInit=[440 55 585 115]  TopName=MinLevel_Right_CAE  DataType=single  BankNumber=0  Role=Automatic
      settings: SourceProductName=Bose Talaria
  TranslateTrigger : TuneVar/TranslateTrigger  TriggerInit=[306 -100 344 -45]
      settings: SourceProductName=Bose Talaria
  Trivial Translation : MATLAB Function  TreatAsAtomicUnit=on
  Tune Variable : TuneVar/Tune Variable  TuneName=MinLevel_Right  SpecifyMaxSize=off  VariableDim=1 (Row)  MaxSize=[1 1]  PackageName=mode  TunabilityNumber=1  MinValue=[0]  MaxValue=[1]  TriggerInit=[-40 25 130 75]  MaskValue=MedusaPremixTune.minGain_Right
      settings: SourceProductName=Bose Talaria
  Out1 : Outport  VectorParamsAs1DForOutWhenUnconnected=off
  Out2 : Outport  Port=2  VectorParamsAs1DForOutWhenUnconnected=off
  wires:
  TOP/1 -> Out1/1  "MinLevel_Right"
  Tune Variable/1 -> Trivial Translation/1(minGain_Right)  "MinLevel_Right"
  Trivial Translation/1(TOP) -> TOP/1
  TranslateTrigger/1 -> Trivial Translation/Trigger
  TOP1/1 -> Out2/1  "MinLevel_Right_CAE"
  Trivial Translation/2(TOP_CAE) -> TOP1/1

== system MedusaPremix/Premix51WithMonoSurroundAndCaeWithFadeRamper/CS Processing/MS Tune ==
  TOP : TOP/TOP  TriggerInit=[260 -150 405 -90]  TopName=Phi  DataType=single  BankNumber=0  Role=Automatic
      settings: SourceProductName=Bose Talaria
  TOP1 : TOP/TOP  TriggerInit=[260 -70 405 -10]  TopName=CosPhi  DataType=single  BankNumber=0  Role=Automatic
      settings: SourceProductName=Bose Talaria
  TOP2 : TOP/TOP  TriggerInit=[260 10 405 70]  TopName=SinPhi  DataType=single  BankNumber=0  Role=Automatic
      settings: SourceProductName=Bose Talaria
  TranslateTrigger : TuneVar/TranslateTrigger  TriggerInit=[66 -245 104 -190]
      settings: SourceProductName=Bose Talaria
  Tune Variable : TuneVar/Tune Variable  TuneName=PhaseAngle  SpecifyMaxSize=off  VariableDim=1 (Row)  MaxSize=[1 1]  PackageName=mode  TunabilityNumber=1  MinValue=[]  MaxValue=[]  TriggerInit=[-270 -65 -100 -15]  MaskValue=MSConfig.DefaultPhaseAngle
      settings: SourceProductName=Bose Talaria
  translation : MATLAB Function  TreatAsAtomicUnit=on
  phi : Outport  VectorParamsAs1DForOutWhenUnconnected=off
  cos(phi) : Outport  Port=2  VectorParamsAs1DForOutWhenUnconnected=off
  sin(phi) : Outport  Port=3  VectorParamsAs1DForOutWhenUnconnected=off
  wires:
  translation/1(phi) -> TOP/1
  TranslateTrigger/1 -> translation/Trigger
  TOP/1 -> phi/1  "Phi"
  Tune Variable/1 -> translation/1(PhaseAngle)  "PhaseAngle"
  translation/2(cos_phi) -> TOP1/1
  TOP1/1 -> cos(phi)/1  "CosPhi"
  translation/3(sin_phi) -> TOP2/1
  TOP2/1 -> sin(phi)/1  "SinPhi"

== system MedusaPremix/Premix51WithMonoSurroundAndCaeWithFadeRamper/CS Processing/Mono-Surround ==
  ChanIn : Inport
  MixCoeff : Inport  Port=2
  Enable : EnablePort
  Add : Sum
  Add1 : Sum  Inputs=+++++
  Concatenation : Concatenate  ConcatenateDimension=2
  Data Store Read : DataStoreRead  DataStoreName=phi  IndexOptions=Index vector (dialog)  Indices=1  OutputSizes=1
  Data Store Read1 : DataStoreRead  DataStoreName=cos_phi  IndexOptions=Index vector (dialog)  Indices=1  OutputSizes=1
  Data Store Read2 : DataStoreRead  DataStoreName=sin_phi  IndexOptions=Index vector (dialog)  Indices=1  OutputSizes=1
  Data Store Read3 : DataStoreRead  DataStoreName=phi  IndexOptions=Index vector (dialog)  Indices=1  OutputSizes=1
  Left Mixer : Subsystem
  Multiply : Product
  Multiply1 : Product
  Right Mixer : Subsystem
  Right Mixer1 : Subsystem
  SOS A : Subsystem
  SOS B : Subsystem
  Selector : Selector  NumberOfDimensions=2  InputPortWidth=10  IndexOptions=Select all,Index vector (dialog)  Indices=[1],1  OutputSizes=1,1
  Selector1 : Selector  NumberOfDimensions=2  InputPortWidth=10  IndexOptions=Select all,Index vector (dialog)  Indices=[2:5],[2:5]  OutputSizes=1,1
  Selector2 : Selector  NumberOfDimensions=2  InputPortWidth=10  IndexOptions=Select all,Index vector (dialog)  Indices=[7:10],[8:11]  OutputSizes=1,1
  Selector3 : Selector  NumberOfDimensions=2  InputPortWidth=10  IndexOptions=Select all,Index vector (dialog)  Indices=[6],[7]  OutputSizes=1,1
  Selector4 : Selector  NumberOfDimensions=2  InputPortWidth=10  IndexOptions=Select all,Index vector (dialog)  Indices=[6],[6 12 13]  OutputSizes=1,1
  Submatrix : matrix_library/Submatrix  RowSpan=All rows  RowStartMode=First  RowStartIndex=1  RowEndMode=Last  RowEndIndex=1  ColSpan=One column  ColStartMode=First  ColStartIndex=1  ColEndMode=Last  ColEndIndex=1
  Submatrix1 : matrix_library/Submatrix  RowSpan=All rows  RowStartMode=First  RowStartIndex=1  RowEndMode=Last  RowEndIndex=1  ColSpan=Range of columns  ColStartMode=Index  ColStartIndex=2  ColEndMode=Index  ColEndIndex=5
  Submatrix2 : matrix_library/Submatrix  RowSpan=All rows  RowStartMode=First  RowStartIndex=1  RowEndMode=Last  RowEndIndex=1  ColSpan=Range of columns  ColStartMode=Index  ColStartIndex=8  ColEndMode=Index  ColEndIndex=11
  Submatrix3 : matrix_library/Submatrix  RowSpan=All rows  RowStartMode=First  RowStartIndex=1  RowEndMode=Last  RowEndIndex=1  ColSpan=One column  ColStartMode=Index  ColStartIndex=7  ColEndMode=Last  ColEndIndex=1
  Submatrix5 : matrix_library/Submatrix  RowSpan=All rows  RowStartMode=First  RowStartIndex=1  RowEndMode=Last  RowEndIndex=1  ColSpan=One column  ColStartMode=Index  ColStartIndex=6  ColEndMode=Last  ColEndIndex=1
  Submatrix6 : matrix_library/Submatrix  RowSpan=All rows  RowStartMode=First  RowStartIndex=1  RowEndMode=Last  RowEndIndex=1  ColSpan=Range of columns  ColStartMode=Index  ColStartIndex=12  ColEndMode=Index  ColEndIndex=13
  cos(phi) : Product
  sin(phi) : Product
  S : Outport  VectorParamsAs1DForOutWhenUnconnected=off
  wires:
  Submatrix/1 -> Multiply/2
  Submatrix1/1 -> Left Mixer/2(MixCoeff)
  Submatrix2/1 -> Right Mixer/2(MixCoeff)
  Submatrix3/1 -> Multiply1/2
  Selector/1 -> Multiply/1  "Lbass"
  Selector1/1 -> Left Mixer/1(AudioIn)  "Lo, Ls, Limp, Ltail"
  Selector2/1 -> Right Mixer/1(AudioIn)  "Ro, Rs, Rimp, Rtail"
  Selector3/1 -> Multiply1/1  "Rbass"
  Right Mixer/1(Output) -> SOS B/1(AudioIn), cos(phi)/2
  cos(phi)/1 -> Add/2
  Left Mixer/1(Output) -> Add/1
  SOS B/1(Out) -> sin(phi)/1
  sin(phi)/1 -> Add1/3
  Multiply1/1 -> Add1/4
  Multiply/1 -> Add1/1
  Add1/1 -> S/1
  SOS A/1(Out) -> Add1/2
  Add/1 -> SOS A/1(AudioIn)
  Data Store Read/1 -> SOS A/2(TuneIn)
  Data Store Read3/1 -> SOS B/2(TuneIn)
  Data Store Read1/1 -> cos(phi)/1
  Data Store Read2/1 -> sin(phi)/2
  MixCoeff/1 -> Submatrix6/1, Submatrix5/1, Submatrix3/1, Submatrix2/1, Submatrix1/1, Submatrix/1
  ChanIn/1 -> Selector/1, Selector1/1, Selector2/1, Selector4/1, Selector3/1
  Selector4/1 -> Right Mixer1/1(AudioIn)  "Lsi, Rsi, Ci"
  Submatrix5/1 -> Concatenation/1
  Submatrix6/1 -> Concatenation/2
  Concatenation/1 -> Right Mixer1/2(MixCoeff)
  Right Mixer1/1(Output) -> Add1/5

== system MedusaPremix/Premix51WithMonoSurroundAndCaeWithFadeRamper/Fade Tuning/Backward Downmix Max ==
  TOP : TOP/TOP  TriggerInit=[440 20 585 80]  TopName=BackwardDownmixMax  DataType=single  BankNumber=0  Role=Automatic
      settings: SourceProductName=Bose Talaria
  TranslateTrigger : TuneVar/TranslateTrigger  TriggerInit=[286 -100 324 -45]
      settings: SourceProductName=Bose Talaria
  Trivial Translation : MATLAB Function  TreatAsAtomicUnit=on
  Tune Variable : TuneVar/Tune Variable  TuneName=BackwardDownmixMax  SpecifyMaxSize=off  VariableDim=1 (Row)  MaxSize=[1 1]  PackageName=mode  TunabilityNumber=1  MinValue=[0]  MaxValue=[1]  TriggerInit=[-65 25 105 75]  MaskValue=MedusaPremixTune.BackwardDownmixMax
      settings: SourceProductName=Bose Talaria
  Out1 : Outport  VectorParamsAs1DForOutWhenUnconnected=off
  wires:
  TranslateTrigger/1 -> Trivial Translation/Trigger
  Trivial Translation/1(TOP) -> TOP/1
  Tune Variable/1 -> Trivial Translation/1(BackwardDownmixMax)  "BackwardDownmixMax"
  TOP/1 -> Out1/1  "BackwardDownmixMax"

== system MedusaPremix/Premix51WithMonoSurroundAndCaeWithFadeRamper/Fade Tuning/Backward Downmix Threshold ==
  TOP : TOP/TOP  TriggerInit=[440 20 585 80]  TopName=BackwardDownmixThreshold  DataType=single  BankNumber=0  Role=Automatic
      settings: SourceProductName=Bose Talaria
  TranslateTrigger : TuneVar/TranslateTrigger  TriggerInit=[306 -100 344 -45]
      settings: SourceProductName=Bose Talaria
  Trivial Translation : MATLAB Function  TreatAsAtomicUnit=on
  Tune Variable : TuneVar/Tune Variable  TuneName=BackwardDownmixThreshold  SpecifyMaxSize=off  VariableDim=1 (Row)  MaxSize=[1 1]  PackageName=mode  TunabilityNumber=1  MinValue=[0]  MaxValue=[1]  TriggerInit=[-75 25 95 75]  MaskValue=MedusaPremixTune.BackwardDownmixThreshold
      settings: SourceProductName=Bose Talaria
  Out1 : Outport  VectorParamsAs1DForOutWhenUnconnected=off
  wires:
  TranslateTrigger/1 -> Trivial Translation/Trigger
  Trivial Translation/1(TOP) -> TOP/1
  Tune Variable/1 -> Trivial Translation/1(BackwardDownmixThreshold)  "BackwardDownmixThreshold"
  TOP/1 -> Out1/1  "BackwardDownmixThreshold"

== system MedusaPremix/Premix51WithMonoSurroundAndCaeWithFadeRamper/Fade Tuning/Downmix Weights CS ==
  TOP : TOP/TOP  TriggerInit=[440 -15 600 45]  TopName=DownmixWeights_CS  DataType=single  BankNumber=0  Role=Automatic
      settings: SourceProductName=Bose Talaria
  TOP1 : TOP/TOP  TriggerInit=[440 55 600 115]  TopName=DownmixWeights_CS_CAE  DataType=single  BankNumber=0  Role=Automatic
      settings: SourceProductName=Bose Talaria
  TranslateTrigger : TuneVar/TranslateTrigger  TriggerInit=[256 -100 294 -45]
      settings: SourceProductName=Bose Talaria
  Trivial Translation : MATLAB Function  TreatAsAtomicUnit=on
  Tune Variable : TuneVar/Tune Variable  TuneName=DownmixWeights_CS  SpecifyMaxSize=off  VariableDim=1 (Row)  MaxSize=[1 1]  PackageName=mode  TunabilityNumber=1  MinValue=[0]  MaxValue=[1]  TriggerInit=[-85 25 85 75]  MaskValue=MedusaPremixTune.downmix_wts_CS
      settings: SourceProductName=Bose Talaria
  Out1 : Outport  VectorParamsAs1DForOutWhenUnconnected=off
  Out2 : Outport  Port=2  VectorParamsAs1DForOutWhenUnconnected=off
  wires:
  Trivial Translation/2(TOP_CAE) -> TOP1/1
  TOP1/1 -> Out2/1  "DownmixWeights_CS_CAE"
  TranslateTrigger/1 -> Trivial Translation/Trigger
  Trivial Translation/1(TOP) -> TOP/1
  Tune Variable/1 -> Trivial Translation/1(downmix_wts_CS)  "DownmixWeights_CS"
  TOP/1 -> Out1/1  "DownmixWeights_CS"

== system MedusaPremix/Premix51WithMonoSurroundAndCaeWithFadeRamper/Fade Tuning/Downmix Weights Left ==
  TOP : TOP/TOP  TriggerInit=[440 -15 605 45]  TopName=DownmixWeights_Left  DataType=single  BankNumber=0  Role=Automatic
      settings: SourceProductName=Bose Talaria
  TOP1 : TOP/TOP  TriggerInit=[440 55 605 115]  TopName=DownmixWeights_Left_CAE  DataType=single  BankNumber=0  Role=Automatic
      settings: SourceProductName=Bose Talaria
  TranslateTrigger : TuneVar/TranslateTrigger  TriggerInit=[266 -100 304 -45]
      settings: SourceProductName=Bose Talaria
  Trivial Translation : MATLAB Function  TreatAsAtomicUnit=on
  Tune Variable : TuneVar/Tune Variable  TuneName=DownmixWeights_Left  SpecifyMaxSize=off  VariableDim=1 (Row)  MaxSize=[1 1]  PackageName=mode  TunabilityNumber=1  MinValue=[0]  MaxValue=[1]  TriggerInit=[-80 25 90 75]  MaskValue=MedusaPremixTune.downmix_wts_Left
      settings: SourceProductName=Bose Talaria
  Out1 : Outport  VectorParamsAs1DForOutWhenUnconnected=off
  Out2 : Outport  Port=2  VectorParamsAs1DForOutWhenUnconnected=off
  wires:
  Trivial Translation/2(TOP_CAE) -> TOP1/1
  TOP1/1 -> Out2/1  "DownmixWeights_Left_CAE"
  TranslateTrigger/1 -> Trivial Translation/Trigger
  Trivial Translation/1(TOP) -> TOP/1
  Tune Variable/1 -> Trivial Translation/1(downmix_wts_Left)  "DownmixWeights_Left"
  TOP/1 -> Out1/1  "DownmixWeights_Left"
